simulink model "PID_drive"  (R2022a)
settings: Solver=VariableStepAuto  StartTime=0.0  StopTime=10.0  RelTol=1e-3
libraries: slpidlib x1
settings Model: SimulationMode=accelerator  Creator=12191  LastModifiedBy=12191

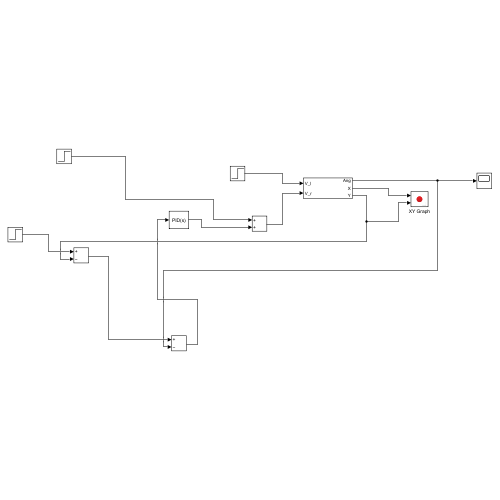
[thumbnail: Simulink's stored preview of the top-level diagram]
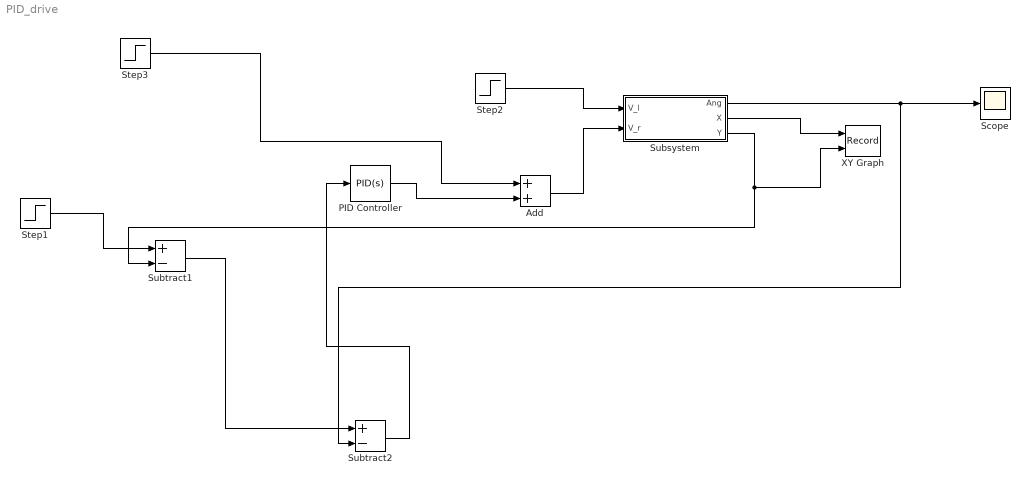
== system PID_drive ==
  Add : Sum
  PID Controller : slpidlib/PID Controller  Controller=PID  Form=Parallel  TimeDomain=Continuous-time  UseExternalTs=off  SampleTime=-1  IntegratorMethod=Forward Euler  FilterMethod=Forward Euler  ControllerParametersSource=internal  P=10  I=8  UseKiTs=off  D=5  N=100  UseFilter=on  TunerSelectOption=Transfer Function Based (PID Tuner App)  InitialConditionSource=internal  InitialConditionForIntegrator=0  InitialConditionForFilter=0  DifferentiatorICPrevScaledInput=0  ExternalReset=none  TrackingMode=off  Kt=1  LimitOutput=off  SatLimitsSource=internal  UpperSaturationLimit=100  LowerSaturationLimit=-100  LinearizeAsGain=on  AntiWindupMode=none  Kb=1  POutMin=[]  POutMax=[]  IOutMin=[]  IOutMax=[]  DOutMin=[]  DOutMax=[]  NOutMin=[]  NOutMax=[]  SumOutMin=[]  SumOutMax=[]  SaturationOutMin=[]  SaturationOutMax=[]  PParamMin=[]  PParamMax=[]  IParamMin=[]  IParamMax=[]  DParamMin=[]  DParamMax=[]  NParamMin=[]  NParamMax=[]  KbParamMin=[]  KbParamMax=[]  KtParamMin=[]  KtParamMax=[]  KbOutMin=[]  KbOutMax=[]  KtOutMin=[]  KtOutMax=[]  IntegratorOutMin=[]  IntegratorOutMax=[]  FilterOutMin=[]  FilterOutMax=[]  SumI1OutMin=[]  SumI1OutMax=[]  SumI2OutMin=[]  SumI2OutMax=[]  SumI3OutMin=[]  SumI3OutMax=[]  SumI4OutMin=[]  SumI4OutMax=[]  SumDOutMin=[]  SumDOutMax=[]  DifferentiatorOutMin=[]  DifferentiatorOutMax=[]  FilterDiffOutCoefMin=[]  FilterDiffOutCoefMax=[]  ReciprocalOutMin=[]  ReciprocalOutMax=[]  SumDenOutMin=[]  SumDenOutMax=[]  SumNumOutMin=[]  SumNumOutMax=[]  DivideOutMin=[]  DivideOutMax=[]  UdiffTsProdOutMin=[]  UdiffTsProdOutMax=[]  NTsProdOutMin=[]  NTsProdOutMax=[]  UintegralTsProdOutMin=[]  UintegralTsProdOutMax=[]  UngainTsProdOutMin=[]  UngainTsProdOutMax=[]  IntegratorContinuousStateAttributes=''  IntegratorStateMustResolveToSignalObject=off  IntegratorRTWStateStorageClass=Auto  FilterContinuousStateAttributes=''  FilterStateMustResolveToSignalObject=off  FilterRTWStateStorageClass=Auto  ParallelPVariant=InternalParameters  IdealPVariant=Disabled  IVariant=InternalParameters  DVariant=InternalParameters  IntegratorVariant=Continuous  SatVariant=Disabled  AWVariant=Passthrough  PCopyVariant=Disabled  TRVariant=Disabled  FdbkBlocksVariant=Forward  IdealPFdbkVariant=Disabled  SatFdbkVariant=Disabled  DerivativeFilterVariant=ContFilter  NVariant=InternalParameters  NCopyVariant=Disabled  FilterICVariant=InternalICsFilter  IntegratorICVariant=InternalICs  ExternalResetVariant=Disabled  TRSumVariant=Passthrough  SumFdbkVariant=Disabled  SumVariant=Sum_PID  TsampFilterVariant=InternalTs  TsampNgainVariant=Passthrough  TsampIntegralVariant=Passthrough  ExternalSaturationOutDataTypeStr=Inherit: Same as second input  aMode=0
  Scope : Scope
  Step1 : Step  Time=2  After=0  SampleTime=0
  Step2 : Step  Time=0  Before=5  After=5  SampleTime=0
  Step3 : Step  Time=0  Before=2  After=2  SampleTime=0
  Subsystem : Subsystem
  Subtract1 : Sum  Inputs=+-
  Subtract2 : Sum  Inputs=+-
  XY Graph : Record  FileSettingsInternal="{\"entries\":[{\"content\":{\"excelSettings\":{\"content\":{},\"type\":\"Streamout.ExcelSettings\"}},\"type\":\"Streamout.FileSettingStorage\",\"uuid\":\"4f2efe64-f4d0-4e2b-bdc5-cae7405f04c4\"}],\"packageUris\":[\"http://schema.mathworks.com/mf0/streamout_blocks/R2020a\"],\"version\":\"1.0\"}"  Layout=[1 1]  SignalsInternal="{\"entries\":[{\"content\":{\"signals\":[{\"content\":{\"blockPath\":[\"PID_drive/XY Graph\"],\"channel\":[],\"dimensions\":[1],\"domain\":\"PID_drive/XY Graph\",\"lineColor\":\"#a2142f\",\"plots\":[1],\"port\":1,\"sid\":[],\"signalID\":29,\"signalName\":\"Subsystem:2\"},\"type\":\"RecordBlkView.Signal\",\"uuid\":\"39bb6528-8c52-4a29-bbde-1edf8c18a79c\"},{\"content\":{\"blockPath\":[\"PID_drive/XY Graph\"],\"channel\":[],\"dimensions\":[1],\"domain\":\"PID_drive/XY Graph\",\"lineColor\":\"#139fff\",\"plots\":[1],\"port\":2,\"sid\":[],\"signalID\":32,\"signalName\":\"Subsystem:3\"},\"type\":\"RecordBlkView.Signal\",\"uuid\":\"261cd562-a94e-4508-bb2d-2b34b34b9b3a\"}]},\"type\":\"RecordBlkView.InputSignals\",\"uuid\":\"53ea45ca-2318-47c1-9695-19c883d68a2a\"}],\"packageUris\":[\"http://schema.mathworks.com/mf0/streamout_blocks/R2020a\"],\"version\":\"1.0\"}"  VisualizationBindings="{\"xyplotplugin\":{\"info\":[{\"series\":[{\"bindingParametersList\":[{\"parameter\":\"X-Axis\",\"signalID\":29,\"signalName\":\"Subsystem:2\"},{\"parameter\":\"Y-Axis\",\"signalID\":32,\"signalName\":\"Subsystem:3\"}],\"seriesID\":48169}],\"subplotID\":1}]}}"  CompatibilityTag=XY
  wires:
  Step1/1 -> Subtract1/1
  Step2/1 -> Subsystem/1(V_l)
  PID Controller/1 -> Add/2
  Step3/1 -> Add/1
  Add/1 -> Subsystem/2(V_r)
  Subsystem/2(X) -> XY Graph/1
  Subsystem/3(Y) -> Subtract1/2, XY Graph/2
  Subsystem/1(Ang) -> Subtract2/2, Scope/1
  Subtract1/1 -> Subtract2/1
  Subtract2/1 -> PID Controller/1

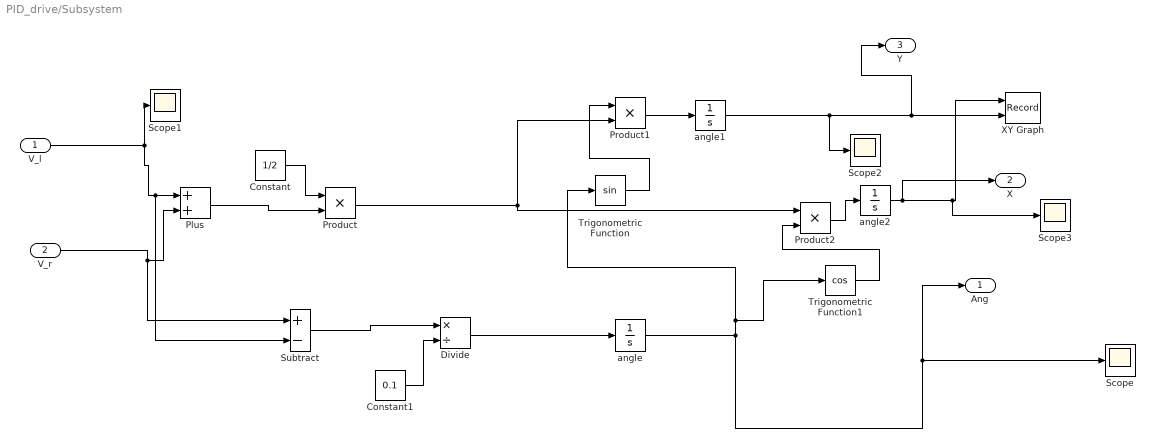
== system PID_drive/Subsystem ==
  V_l : Inport
  V_r : Inport  Port=2
  Constant : Constant  Value=1/2
  Constant1 : Constant  Value=0.1
  Divide : Product  Inputs=*/
  Plus : Sum
  Product : Product
  Product1 : Product
  Product2 : Product
  Scope{,1..3} (4 alike) : Scope
  Subtract : Sum  Inputs=+-
  Trigonometric Function : Trigonometry
  Trigonometric Function1 : Trigonometry  Operator=cos
  XY Graph : Record  FileSettingsInternal="{\"entries\":[{\"content\":{\"excelSettings\":{\"content\":{},\"type\":\"Streamout.ExcelSettings\"}},\"type\":\"Streamout.FileSettingStorage\",\"uuid\":\"2e562e4a-e3dc-4566-ac71-ed3ae64635fc\"}],\"packageUris\":[\"http://schema.mathworks.com/mf0/streamout_blocks/R2020a\"],\"version\":\"1.0\"}"  Layout=[1 1]  SignalsInternal="{\"entries\":[{\"content\":{\"signals\":[{\"content\":{\"blockPath\":[\"PID_drive/Subsystem/XY Graph\"],\"channel\":[],\"dimensions\":[1],\"domain\":\"PID_drive/Subsystem/XY Graph\",\"lineColor\":\"#edb120\",\"plots\":[],\"port\":1,\"sid\":[],\"signalID\":37,\"signalName\":\"angle2\"},\"type\":\"RecordBlkView.Signal\",\"uuid\":\"91fc224c-6dcd-4385-906d-8f882d445a3a\"},{\"content\":{\"blockPath\":[\"PID_drive/Subsystem/XY Graph\"],\"channel\":[],\"dimensions\":[1],\"domain\":\"PID_drive/Subsystem/XY Graph\",\"lineColor\":\"#7e2f8e\",\"plots\":[],\"port\":2,\"sid\":[],\"signalID\":40,\"signalName\":\"angle1\"},\"type\":\"RecordBlkView.Signal\",\"uuid\":\"37f00c99-2566-4220-b66d-57b2a772e07d\"}]},\"type\":\"RecordBlkView.InputSignals\",\"uuid\":\"badf5347-3999-496e-b885-d6c6441dda7c\"}],\"packageUris\":[\"http://schema.mathworks.com/mf0/streamout_blocks/R2020a\"],\"version\":\"1.0\"}"  VisualizationBindings="{\"sparklinesplugin\":{\"info\":[{\"bindingParametersList\":[],\"subplotID\":1}]}}"  CompatibilityTag=XY
  angle : Integrator
  angle1 : Integrator
  angle2 : Integrator
  Ang : Outport
  X : Outport  Port=2
  Y : Outport  Port=3
  wires:
  Constant1/1 -> Divide/2
  Subtract/1 -> Divide/1
  Constant/1 -> Product/1
  V_r/1 -> Subtract/1, Plus/2
  Divide/1 -> angle/1
  angle2/1 -> X/1, Scope3/1, XY Graph/1
  Product/1 -> Product2/1, Product1/2
  Plus/1 -> Product/2
  Trigonometric Function/1 -> Product1/1
  V_l/1 -> Subtract/2, Plus/1, Scope1/1
  Product2/1 -> angle2/1
  Trigonometric Function1/1 -> Product2/2
  angle1/1 -> Scope2/1, Y/1, XY Graph/2
  Product1/1 -> angle1/1
  angle/1 -> Trigonometric Function/1, Trigonometric Function1/1, Scope/1, Ang/1
